simulink model "HasenFuexse"  (Simulink 7.7)
settings: Solver=ode45  StartTime=0.0  StopTime=10.0  RelTol=1e-3
settings Model: Creator=hexren  LastModifiedBy=hexren

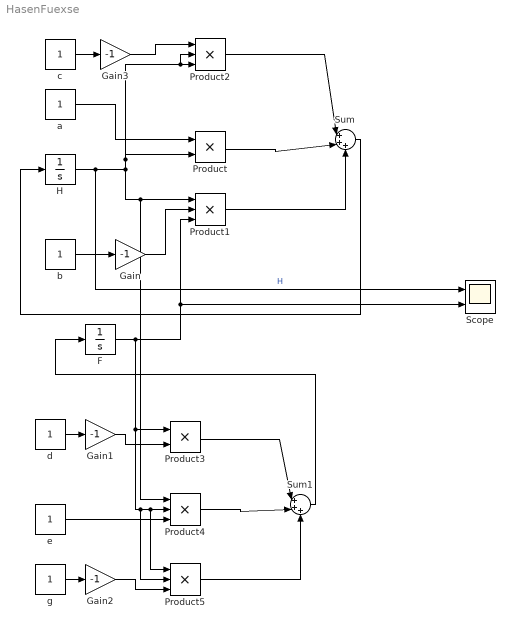
== system HasenFuexse ==
  F : Integrator  InitialCondition=2
  Gain{,1..3} (4 alike) : Gain  Gain=-1
  H : Integrator  InitialCondition=10
  Product : Product  RndMeth=Zero
  Product{1..2,4..5} (4 alike) : Product  Inputs=3  RndMeth=Zero
  Product3 : Product  RndMeth=Zero
  Scope : Scope  NumInputPorts=2
      settings: YMin=-5~-5  YMax=5~5
  Sum : Sum  Inputs=|+++
  Sum1 : Sum  Inputs=|+++
  a : Constant
  b : Constant
  c : Constant
  d : Constant
  e : Constant
  g : Constant
  wires:
  a/1 -> Product/1
  H/1 -> Product/2, Product2/2, Product2/3, Product1/1, Product4/1, Scope/1  "H"
  b/1 -> Gain/1
  Gain/1 -> Product1/2
  F/1 -> Product3/1, Product4/2, Product5/1, Product5/2, Product1/3, Scope/2
  Product/1 -> Sum/2
  Product2/1 -> Sum/1
  Product1/1 -> Sum/3
  Sum/1 -> H/1
  d/1 -> Gain1/1
  Gain1/1 -> Product3/2
  e/1 -> Product4/3
  g/1 -> Gain2/1
  Gain2/1 -> Product5/3
  Product3/1 -> Sum1/1
  Product4/1 -> Sum1/2
  Product5/1 -> Sum1/3
  Sum1/1 -> F/1
  c/1 -> Gain3/1
  Gain3/1 -> Product2/1
